simulink model "baseline_controller"  (R2023b)
settings: Solver=VariableStepAuto  StartTime=0.0  StopTime=10.0  RelTol=1e-3
settings Model: Creator=fabioschneider  LastModifiedBy=fabioschneider

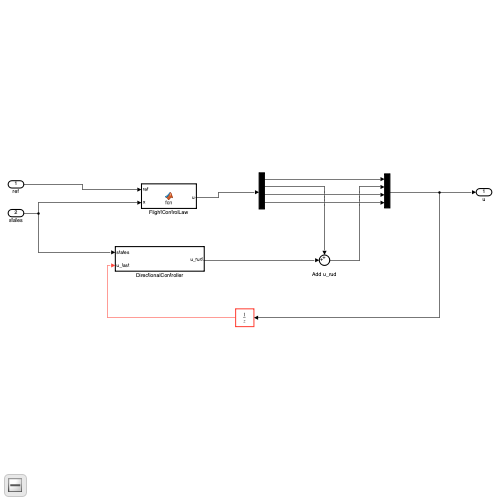
[thumbnail: Simulink's stored preview of the top-level diagram]
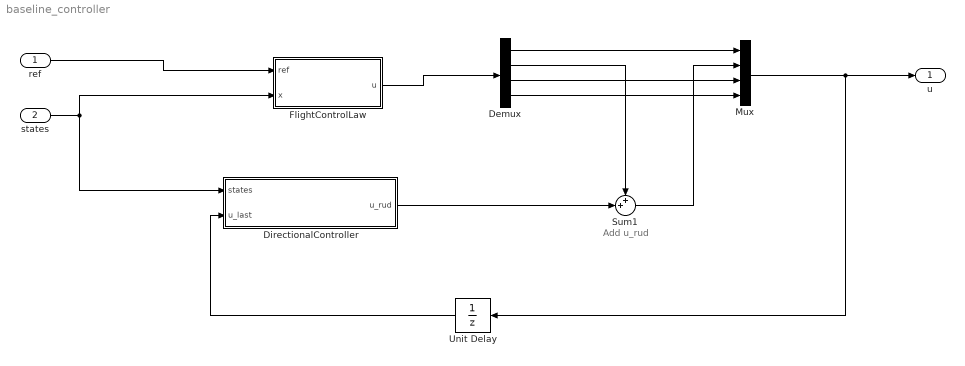
== system baseline_controller ==
  note: Add u_rud
  ref : Inport  PortDimensions=4
  states : Inport  Port=2
  Demux : Demux
  DirectionalController : Subsystem
  FlightControlLaw : MATLAB Function  TreatAsAtomicUnit=on
  Mux : Mux
  Sum1 : Sum  Inputs=++|
  Unit Delay : UnitDelay  InitialCondition=[0;0;0;14500]  SampleTime=-1  HasFrameUpgradeWarning=on
  u : Outport
  wires:
  Demux/1 -> Mux/1
  Demux/2 -> Sum1/1
  Sum1/1 -> Mux/2
  Demux/4 -> Mux/4
  DirectionalController/1(u_rud) -> Sum1/2
  Mux/1 -> Unit Delay/1, u/1
  FlightControlLaw/1(u) -> Demux/1
  Demux/3 -> Mux/3
  states/1 -> DirectionalController/1(states), FlightControlLaw/2(x)
  ref/1 -> FlightControlLaw/1(ref)
  Unit Delay/1 -> DirectionalController/2(u_last)

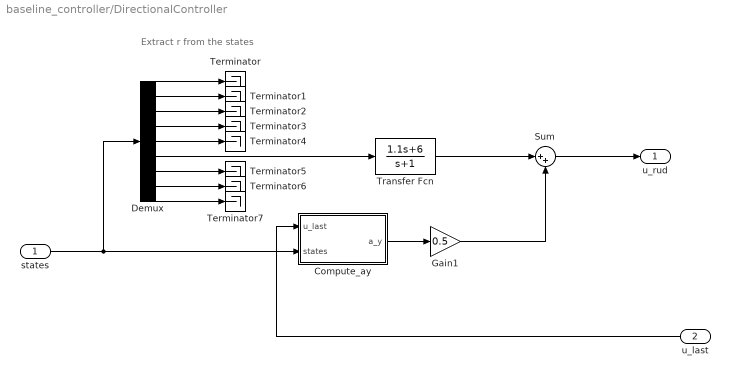
== system baseline_controller/DirectionalController ==
  note: Extract r from the states
  states : Inport
  u_last : Inport  Port=2
  Compute_ay : MATLAB Function  TreatAsAtomicUnit=on
  Demux : Demux  Outputs=9
  Gain1 : Gain  Gain=0.5
  Sum : Sum  Inputs=|++
  Terminator{,1..7} (8 alike) : Terminator
  Transfer Fcn : TransferFcn  Numerator=[1.1, 6]  Denominator=[1 1]
  u_rud : Outport
  wires:
  Sum/1 -> u_rud/1
  states/1 -> Compute_ay/2(states), Demux/1
  Compute_ay/1(a_y) -> Gain1/1
  Demux/6 -> Transfer Fcn/1
  Transfer Fcn/1 -> Sum/1
  u_last/1 -> Compute_ay/1(u_last)
  Gain1/1 -> Sum/2
  Demux/1 -> Terminator/1
  Demux/2 -> Terminator1/1
  Demux/3 -> Terminator2/1
  Demux/4 -> Terminator3/1
  Demux/5 -> Terminator4/1
  Demux/7 -> Terminator5/1
  Demux/8 -> Terminator6/1
  Demux/9 -> Terminator7/1

== matlab function baseline_controller/FlightControlLaw ==
  data: ref input; u output size=[4, 1]; x input
function u = fcn(ref, x)
    % INPUT:
    %   ref = [ustab; urud; uail; uthr] Reference input signal
    %   x = [Velocity; sideslip_angle; angle_of_attack; rool_rate; pitch_rate; 
    %        yaw_rate; bank_angle; pitch_angle; yaw_angle]
    % OUTPUT:
    %   u = [ustab; urud; uail; uthr] Input signal for plant
    u = baseline_control_law(ref,x);

== matlab function baseline_controller/DirectionalController/Compute_ay ==
  data: u_last input; a_y output; states input
function a_y = fcn(u_last,states)
    % INPUT:
    %   u_last = [ustab; urud; uail; uthr] input signal from last
    %   simulation step
    %   states = [Velocity; sideslip_angle; angle_of_attack; rool_rate; pitch_rate; 
    %        yaw_rate; bank_angle; pitch_angle; yaw_angle]
    % OUTPUT:
    %   a_y normal accelearation along the y axi


    a_y = compute_ay(u_last, states);
